simulink model "lab1_5"  (R2020a)
settings: Solver=VariableStepAuto  StartTime=0.0  StopTime=10.0  RelTol=1e-3
settings Model: Creator=huang  LastModifiedBy=huang

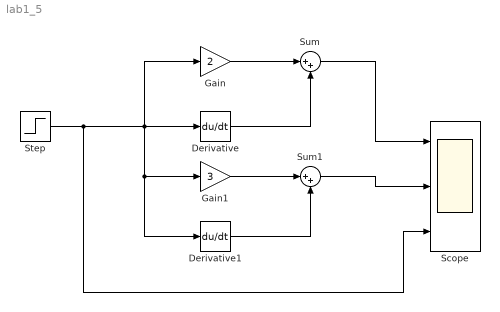
== system lab1_5 ==
  Derivative : Derivative  CoefficientInTFapproximation=1/20
  Derivative1 : Derivative  CoefficientInTFapproximation=1/15
  Gain : Gain  Gain=2
  Gain1 : Gain  Gain=3
  Scope : Scope  NumInputPorts=3
  Step : Step  Time=0  SampleTime=0
  Sum : Sum  Inputs=|++
  Sum1 : Sum  Inputs=|++
  wires:
  Gain/1 -> Sum/1
  Derivative/1 -> Sum/2
  Sum/1 -> Scope/1
  Step/1 -> Scope/3, Derivative/1, Derivative1/1, Gain1/1, Gain/1
  Derivative1/1 -> Sum1/2
  Gain1/1 -> Sum1/1
  Sum1/1 -> Scope/2
